simulink model "CDHRM_model_v1"  (R2019b)
settings: Solver=VariableStepAuto  StartTime=0.0  StopTime=10.0  RelTol=1e-3
InitFcn:
  | parameters.m
values from neighbouring files (symbols this model uses):
  a = 140/1000    (= 0.14)    [parameters.m]
  d = 23/2000    (= 0.0115)    [parameters.m]
  eta = 0.39    [parameters.m]
  g = 9.81    [parameters.m]
  J_L = 0.014 * 10e-7    (= 1.4e-08)    [parameters.m]
  J_R = 0.864 * 10e-7    (= 8.64e-07)    [parameters.m]
  k_m = 2560*100*pi/3    (= 268082.573106)    [parameters.m]
  k_trans = 0.36    [parameters.m]
  l_link = a-2*d    (= 0.117)    [parameters.m]
  m = 0.2    [parameters.m]
  mu_cable = 0.17    [parameters.m]
  n_0 = 9620*pi/30    (= 1007.40404425)    [parameters.m]
  p = 8/1000    (= 0.008)    [parameters.m]
  r = 20.5/1000    (= 0.0205)    [parameters.m]
  r_drum = 0.042    [parameters.m]
undefined symbols (not defined in the file or in its folder): d_drum
libraries: dspindex x18, dspinverses x1, simulink x1
(part 4 of 5)

== matlab function CDHRM_model_v1/Dynamic Model of the arm/M_inv(theta)/Newton-Euler Inverse Dynamics Block 11/Newton-Euler Recursive Inverse Dynamics Block ==
  data: theta input; u output; d_theta input; dd_theta input; m input; a input; d input; r input; g input; F_ec input; T_ec input
%% Neton-Euler Recursive Algorithm for Inverse Dynamics
function u  = fcn(theta, d_theta,dd_theta,m,a,d,r,g,F_ec,T_ec)
%% Parameters
N=9;
P_joint_to_joint=[a+2*d;0;0];
P_link_cm=[-(a/2+d);0;0];
z_0=[0;0;1];
x_0=[1;0;0];
% Create the D-H parameter table
DH_params=zeros(2*N,4);
for i=1:N
    if rem(i,2)==0
        DH_params(2*i-1:2*i,:)=[180+(theta(2*i-1)*180/pi) 90 0 0;...
                                180+(theta(2*i)*180/pi) 0 a 0];
    else
        DH_params(2*i-1:2*i,:)=[theta(2*i-1)*180/pi 90 0 0;...
                                theta(2*i)*180/pi 0 a 0];
    end
end
% Calculate transformation matrix n_A_n+1 (A_wrt_prev) and store in cell
% array
R = cell(2*N,1);
for n=1:2*N
    theta_i=DH_params(n,1);
    alpha_i=DH_params(n,2);
    R{n}=[cosd(theta_i) -sind(theta_i)*cosd(alpha_i) sind(theta_i)*sind(alpha_i);...
       sind(theta_i)  cosd(theta_i)*cosd(alpha_i) -cosd(theta_i)*sind(alpha_i);...
                  0              sind(alpha_i)   cosd(alpha_i) ];
end
% Calculate Inertia tensor
I = cell(N,1);
for i=1:N
    I{i}=[1/12*(m*(a)^2)+1/4*(m*r^2) 0 0;
                      0 1/12*(m*(a)^2)+1/4*(m*r^2) 0;
                      0 0 1/4*(m*r^2)];
end
%% Forward recursion
% Initialising the matrices
omega=zeros(3,N);
d_omega=zeros(3,N);
a_joint=zeros(3,N);
a_c=zeros(3,N);
% Initialising prev values
omega_prev=zeros(3,1);
d_omega_prev=zeros(3,1);
a_joint_prev=zeros(3,1);
for n=1:N
    omega(:,n)=(R{2*n-1}*R{2*n})'*(omega_prev + z_0*d_theta(2*n-1)) + ...
               (R{2*n})'*z_0*d_theta(2*n);
    d_omega(:,n)=(R{2*n-1}*R{2*n})'*(d_omega_prev + z_0*dd_theta(2*n-1)+...
                                     cross(omega(:,n),z_0*d_theta(2*n-1))) + ...
                 (R{2*n-1}*R{2*n})'*(cross((z_0*d_theta(2*n-1) + omega_prev),R{2*n-1}*z_0*d_theta(2*n))) + ...
                 (R{2*n})'*(z_0*dd_theta(2*n));
    if n==1
        a_joint(:,n)=[0;0;g];
    else
        a_joint(:,n)=(R{2*n-3}*R{2*n-2})'*a_joint_prev+ ...
                     cross(d_omega_prev,P_joint_to_joint)+...
                     cross(omega_prev,cross(omega_prev,P_joint_to_joint));
    end
    a_c(:,n)=(R{2*n-1}*R{2*n})'*a_joint(:,n)+...
             cross(d_omega(:,n),(P_joint_to_joint+P_link_cm))+...
             cross(omega(:,n),cross(omega(:,n),(P_joint_to_joint+P_link_cm)));
    % Update prev values for next iteration
    omega_prev=omega(:,n);
    d_omega_prev=d_omega(:,n);
    a_joint_prev=a_joint(:,n);
end

%% Backward recursion
% Initialising the matrices
F=zeros(3,N);
tau=zeros(3,N);
% Initialise next values
F_next=zeros(3,1);
tau_next=zeros(3,1);
for n=N:-1:1
   F(:,n) = F_next + m*a_c(:,n)-F_ec(:,n);
   tau(:,n) = tau_next - cross(F(:,n),(P_joint_to_joint+P_link_cm)) + ...
              cross(F_next,P_link_cm) + ...
              I{n}*d_omega(:,n)+ cross(omega(:,n),I{n}*omega(:,n))-T_ec(:,n);
   % Update next values for next iteration
   F_next=F(:,n);
   tau_next=tau(:,n);
end
%% Computing the output
u=vecnorm(tau)';

== matlab function CDHRM_model_v1/Dynamic Model of the arm/M_inv(theta)/Newton-Euler Inverse Dynamics Block 12/Cable Contact Forces ==
  data: tau_m input; theta input; a input; d input; r input; F_ec output; T_ec output; r_drum input; l_link input; eta input; mu input
function [F_ec,T_ec] = fcn(tau_m,theta,a,d,r,r_drum, l_link,eta,mu)
N=9;
F_ec=zeros(3,N);
T_ec=zeros(3,N);
F_cd=cell(N,3*N);
F_cp=cell(N,3*N);
for i=1:N
    for j=1:3*N
        F_cd{i,j}=[0;0;0];
        F_cp{i,j}=[0;0;0]; 
    end
end
r_d=cell(N,3*N);
r_p=cell(N,3*N);
T_p=cell(N,3*N);
T_d=cell(N,3*N);
P_link_cm=[-(a/2+d);0;0];
% Initialise prev values
Td_0=tau_m*r_drum/eta;
% Calculate the Transformation matrices
DH_params=zeros(2*N,4);
for i=1:N
    if rem(i,2)==0
        DH_params(2*i-1:2*i,:)=[180+(theta(2*i-1)*180/pi) 90 0 0; 180+(theta(2*i)*180/pi) 0 a 0];
    else
        DH_params(2*i-1:2*i,:)=[(theta(2*i-1)*180/pi) 90 0 0; (theta(2*i)*180/pi) 0 a 0];
    end
end

% Calculate transformation matrix n_A_n+1 (A_wrt_prev) and store in cell
% array
A = cell(2*N,1);
for n=1:2*N
    theta_i=DH_params(n,1);
    alpha_i=DH_params(n,2);
    r_i=DH_params(n,3);
    d_i=DH_params(n,4);
    A{n}=[cosd(theta_i) -sind(theta_i)*cosd(alpha_i) sind(theta_i)*sind(alpha_i) r_i*cosd(theta_i);...
       sind(theta_i)  cosd(theta_i)*cosd(alpha_i) -cosd(theta_i)*sind(alpha_i) r_i*sind(theta_i);...
                  0              sind(alpha_i)   cosd(alpha_i)              d_i;...
                  0              0              0                         1];
end

% Create a list of transformation matrices wrt base for all joints
A_wrt_base=cell(2*N,1);
A_wrt_base{1}=A{1};
for n=2:2*N
    A_wrt_base{n}=A_wrt_base{n-1}*A{n};
end

for i=1:N
    for j=1:3*N
        M=floor((j-1)/3)+1;
        if j==1
           Td_prev=Td_0(j);
        end
        % Calculate delta and r
        if rem(i,2)==0
            delta_p=((120/(N+1))*(M)+120*(j-1)+87);
            delta_d=((120/(N+1))*(M)+120*(j-1)-3);
            r_p_j=[d-l_link; r*cosd(delta_p);r*sind(delta_p); 1];
            r_d_j=[-d;r*cosd(delta_d);r*sind(delta_d); 1];
        else
            delta_p=((120/(N+1))*(M)+120*(j-1)-3);
            delta_d=((120/(N+1))*(M)+120*(j-1)+87);
            if i==1
                L_d_prev=[-d;r*cosd(delta_d);r*sind(delta_d); 1];
                e_d_prev=L_d_prev(1:3)/norm(L_d_prev(1:3));
                e_d_0=e_d_prev;
                r_d_prev=[-d;r*cosd(delta_d);r*sind(delta_d); 1];
            end
            r_p_j=[d-l_link; r*sind(delta_p);-r*cosd(delta_p); 1];
            r_d_j=[-d;r*sind(delta_d);-r*cosd(delta_d); 1];
        end
        r_p{i,j}=r_p_j(1:3);
        r_d{i,j}=r_d_j(1:3);
        % Calculate L
        if i==1
            L_p=(A{2*i}*r_p_j)-(r_d_prev);
        else
            L_p=(A{2*i}*r_p_j)-(A{2*i-2}*r_d_prev);
        end
        L_d=A{2*i}*(r_d_j-r_p_j);
        % Calculate e
        e_p=L_p(1:3)/norm(L_p(1:3));
        e_d=L_d(1:3)/norm(L_d(1:3));
        % Calculate phi
        phi_p=acos(dot(e_p,e_d));
        phi_d=acos(dot(e_d_prev,e_p));
        % Get Tp
        T_p_j=Td_prev/(exp(mu*phi_d));
        T_p{i,j}=T_p_j*e_p;
        % Get Td
        T_d_j=T_p_j/(exp(mu*phi_p));
        T_d{i,j}=T_d_j*e_d;
        % Update prev values
        e_d_prev=e_d;
        r_d_prev=r_d_j;
        Td_prev=T_d_j;
    end
end

% Calculate F_cp and F_cd
for n=1:N
    for k=1:3*N
        M=floor((k-1)/3)+1;
        if (3*n+1 <= k) && (k<=3*N) && n<=M
            F_cp{n,k}=T_d{n,k}-T_p{n,k};
            if n==1
                F_cd{n,k}=T_p{n,k}-((tau_m(k)*r_drum/eta)*e_d_0);
            else
                F_cd{n,k}=T_p{n,k}-T_d{n-1,k};
            end
        end
        if (3*n-2 <= k) && (k <=3*n) && n==M
            F_cp{n,k}=-T_p{n,k};
        end
    end
end

% Calculate F_ec
for n=1:N
    F_ec_n=[0;0;0];
    A_2n=inv(A{2*n});
    R_2n=A_2n(1:3,1:3);
    for k=3*n+1:3*N
        F_ec_n=F_ec_n+((R_2n)*F_cd{n,k});
    end
    for k=3*n-2:3*N
        F_ec_n=F_ec_n+((R_2n)*F_cp{n,k});
    end
    F_ec(:,n)=F_ec_n;
end

% Calculate T_ec
for n=1:N
    T_ec_n=[0;0;0];
    A_2n=inv(A{2*n});
    R_2n=A_2n(1:3,1:3);
    for k=3*n+1:3*N
        T_ec_n=T_ec_n+cross((r_d{n,k}-P_link_cm),((R_2n)*F_cd{n,k}));
    end
    for k=3*n-2:3*N
        T_ec_n=T_ec_n+cross((r_p{n,k}-P_link_cm),((R_2n)*F_cp{n,k}));
    end
    T_ec(:,n)=T_ec_n;
end

== matlab function CDHRM_model_v1/Dynamic Model of the arm/M_inv(theta)/Newton-Euler Inverse Dynamics Block 12/Newton-Euler Recursive Inverse Dynamics Block ==
  data: theta input; u output; d_theta input; dd_theta input; m input; a input; d input; r input; g input; F_ec input; T_ec input
%% Neton-Euler Recursive Algorithm for Inverse Dynamics
function u  = fcn(theta, d_theta,dd_theta,m,a,d,r,g,F_ec,T_ec)
%% Parameters
N=9;
P_joint_to_joint=[a+2*d;0;0];
P_link_cm=[-(a/2+d);0;0];
z_0=[0;0;1];
x_0=[1;0;0];
% Create the D-H parameter table
DH_params=zeros(2*N,4);
for i=1:N
    if rem(i,2)==0
        DH_params(2*i-1:2*i,:)=[180+(theta(2*i-1)*180/pi) 90 0 0;...
                                180+(theta(2*i)*180/pi) 0 a 0];
    else
        DH_params(2*i-1:2*i,:)=[theta(2*i-1)*180/pi 90 0 0;...
                                theta(2*i)*180/pi 0 a 0];
    end
end
% Calculate transformation matrix n_A_n+1 (A_wrt_prev) and store in cell
% array
R = cell(2*N,1);
for n=1:2*N
    theta_i=DH_params(n,1);
    alpha_i=DH_params(n,2);
    R{n}=[cosd(theta_i) -sind(theta_i)*cosd(alpha_i) sind(theta_i)*sind(alpha_i);...
       sind(theta_i)  cosd(theta_i)*cosd(alpha_i) -cosd(theta_i)*sind(alpha_i);...
                  0              sind(alpha_i)   cosd(alpha_i) ];
end
% Calculate Inertia tensor
I = cell(N,1);
for i=1:N
    I{i}=[1/12*(m*(a)^2)+1/4*(m*r^2) 0 0;
                      0 1/12*(m*(a)^2)+1/4*(m*r^2) 0;
                      0 0 1/4*(m*r^2)];
end
%% Forward recursion
% Initialising the matrices
omega=zeros(3,N);
d_omega=zeros(3,N);
a_joint=zeros(3,N);
a_c=zeros(3,N);
% Initialising prev values
omega_prev=zeros(3,1);
d_omega_prev=zeros(3,1);
a_joint_prev=zeros(3,1);
for n=1:N
    omega(:,n)=(R{2*n-1}*R{2*n})'*(omega_prev + z_0*d_theta(2*n-1)) + ...
               (R{2*n})'*z_0*d_theta(2*n);
    d_omega(:,n)=(R{2*n-1}*R{2*n})'*(d_omega_prev + z_0*dd_theta(2*n-1)+...
                                     cross(omega(:,n),z_0*d_theta(2*n-1))) + ...
                 (R{2*n-1}*R{2*n})'*(cross((z_0*d_theta(2*n-1) + omega_prev),R{2*n-1}*z_0*d_theta(2*n))) + ...
                 (R{2*n})'*(z_0*dd_theta(2*n));
    if n==1
        a_joint(:,n)=[0;0;g];
    else
        a_joint(:,n)=(R{2*n-3}*R{2*n-2})'*a_joint_prev+ ...
                     cross(d_omega_prev,P_joint_to_joint)+...
                     cross(omega_prev,cross(omega_prev,P_joint_to_joint));
    end
    a_c(:,n)=(R{2*n-1}*R{2*n})'*a_joint(:,n)+...
             cross(d_omega(:,n),(P_joint_to_joint+P_link_cm))+...
             cross(omega(:,n),cross(omega(:,n),(P_joint_to_joint+P_link_cm)));
    % Update prev values for next iteration
    omega_prev=omega(:,n);
    d_omega_prev=d_omega(:,n);
    a_joint_prev=a_joint(:,n);
end

%% Backward recursion
% Initialising the matrices
F=zeros(3,N);
tau=zeros(3,N);
% Initialise next values
F_next=zeros(3,1);
tau_next=zeros(3,1);
for n=N:-1:1
   F(:,n) = F_next + m*a_c(:,n)-F_ec(:,n);
   tau(:,n) = tau_next - cross(F(:,n),(P_joint_to_joint+P_link_cm)) + ...
              cross(F_next,P_link_cm) + ...
              I{n}*d_omega(:,n)+ cross(omega(:,n),I{n}*omega(:,n))-T_ec(:,n);
   % Update next values for next iteration
   F_next=F(:,n);
   tau_next=tau(:,n);
end
%% Computing the output
u=vecnorm(tau)';

== matlab function CDHRM_model_v1/Dynamic Model of the arm/M_inv(theta)/Newton-Euler Inverse Dynamics Block 13/Cable Contact Forces ==
  data: tau_m input; theta input; a input; d input; r input; F_ec output; T_ec output; r_drum input; l_link input; eta input; mu input
function [F_ec,T_ec] = fcn(tau_m,theta,a,d,r,r_drum, l_link,eta,mu)
N=9;
F_ec=zeros(3,N);
T_ec=zeros(3,N);
F_cd=cell(N,3*N);
F_cp=cell(N,3*N);
for i=1:N
    for j=1:3*N
        F_cd{i,j}=[0;0;0];
        F_cp{i,j}=[0;0;0]; 
    end
end
r_d=cell(N,3*N);
r_p=cell(N,3*N);
T_p=cell(N,3*N);
T_d=cell(N,3*N);
P_link_cm=[-(a/2+d);0;0];
% Initialise prev values
Td_0=tau_m*r_drum/eta;
% Calculate the Transformation matrices
DH_params=zeros(2*N,4);
for i=1:N
    if rem(i,2)==0
        DH_params(2*i-1:2*i,:)=[180+(theta(2*i-1)*180/pi) 90 0 0; 180+(theta(2*i)*180/pi) 0 a 0];
    else
        DH_params(2*i-1:2*i,:)=[(theta(2*i-1)*180/pi) 90 0 0; (theta(2*i)*180/pi) 0 a 0];
    end
end

% Calculate transformation matrix n_A_n+1 (A_wrt_prev) and store in cell
% array
A = cell(2*N,1);
for n=1:2*N
    theta_i=DH_params(n,1);
    alpha_i=DH_params(n,2);
    r_i=DH_params(n,3);
    d_i=DH_params(n,4);
    A{n}=[cosd(theta_i) -sind(theta_i)*cosd(alpha_i) sind(theta_i)*sind(alpha_i) r_i*cosd(theta_i);...
       sind(theta_i)  cosd(theta_i)*cosd(alpha_i) -cosd(theta_i)*sind(alpha_i) r_i*sind(theta_i);...
                  0              sind(alpha_i)   cosd(alpha_i)              d_i;...
                  0              0              0                         1];
end

% Create a list of transformation matrices wrt base for all joints
A_wrt_base=cell(2*N,1);
A_wrt_base{1}=A{1};
for n=2:2*N
    A_wrt_base{n}=A_wrt_base{n-1}*A{n};
end

for i=1:N
    for j=1:3*N
        M=floor((j-1)/3)+1;
        if j==1
           Td_prev=Td_0(j);
        end
        % Calculate delta and r
        if rem(i,2)==0
            delta_p=((120/(N+1))*(M)+120*(j-1)+87);
            delta_d=((120/(N+1))*(M)+120*(j-1)-3);
            r_p_j=[d-l_link; r*cosd(delta_p);r*sind(delta_p); 1];
            r_d_j=[-d;r*cosd(delta_d);r*sind(delta_d); 1];
        else
            delta_p=((120/(N+1))*(M)+120*(j-1)-3);
            delta_d=((120/(N+1))*(M)+120*(j-1)+87);
            if i==1
                L_d_prev=[-d;r*cosd(delta_d);r*sind(delta_d); 1];
                e_d_prev=L_d_prev(1:3)/norm(L_d_prev(1:3));
                e_d_0=e_d_prev;
                r_d_prev=[-d;r*cosd(delta_d);r*sind(delta_d); 1];
            end
            r_p_j=[d-l_link; r*sind(delta_p);-r*cosd(delta_p); 1];
            r_d_j=[-d;r*sind(delta_d);-r*cosd(delta_d); 1];
        end
        r_p{i,j}=r_p_j(1:3);
        r_d{i,j}=r_d_j(1:3);
        % Calculate L
        if i==1
            L_p=(A{2*i}*r_p_j)-(r_d_prev);
        else
            L_p=(A{2*i}*r_p_j)-(A{2*i-2}*r_d_prev);
        end
        L_d=A{2*i}*(r_d_j-r_p_j);
        % Calculate e
        e_p=L_p(1:3)/norm(L_p(1:3));
        e_d=L_d(1:3)/norm(L_d(1:3));
        % Calculate phi
        phi_p=acos(dot(e_p,e_d));
        phi_d=acos(dot(e_d_prev,e_p));
        % Get Tp
        T_p_j=Td_prev/(exp(mu*phi_d));
        T_p{i,j}=T_p_j*e_p;
        % Get Td
        T_d_j=T_p_j/(exp(mu*phi_p));
        T_d{i,j}=T_d_j*e_d;
        % Update prev values
        e_d_prev=e_d;
        r_d_prev=r_d_j;
        Td_prev=T_d_j;
    end
end

% Calculate F_cp and F_cd
for n=1:N
    for k=1:3*N
        M=floor((k-1)/3)+1;
        if (3*n+1 <= k) && (k<=3*N) && n<=M
            F_cp{n,k}=T_d{n,k}-T_p{n,k};
            if n==1
                F_cd{n,k}=T_p{n,k}-((tau_m(k)*r_drum/eta)*e_d_0);
            else
                F_cd{n,k}=T_p{n,k}-T_d{n-1,k};
            end
        end
        if (3*n-2 <= k) && (k <=3*n) && n==M
            F_cp{n,k}=-T_p{n,k};
        end
    end
end

% Calculate F_ec
for n=1:N
    F_ec_n=[0;0;0];
    A_2n=inv(A{2*n});
    R_2n=A_2n(1:3,1:3);
    for k=3*n+1:3*N
        F_ec_n=F_ec_n+((R_2n)*F_cd{n,k});
    end
    for k=3*n-2:3*N
        F_ec_n=F_ec_n+((R_2n)*F_cp{n,k});
    end
    F_ec(:,n)=F_ec_n;
end

% Calculate T_ec
for n=1:N
    T_ec_n=[0;0;0];
    A_2n=inv(A{2*n});
    R_2n=A_2n(1:3,1:3);
    for k=3*n+1:3*N
        T_ec_n=T_ec_n+cross((r_d{n,k}-P_link_cm),((R_2n)*F_cd{n,k}));
    end
    for k=3*n-2:3*N
        T_ec_n=T_ec_n+cross((r_p{n,k}-P_link_cm),((R_2n)*F_cp{n,k}));
    end
    T_ec(:,n)=T_ec_n;
end

== matlab function CDHRM_model_v1/Dynamic Model of the arm/M_inv(theta)/Newton-Euler Inverse Dynamics Block 13/Newton-Euler Recursive Inverse Dynamics Block ==
  data: theta input; u output; d_theta input; dd_theta input; m input; a input; d input; r input; g input; F_ec input; T_ec input
%% Neton-Euler Recursive Algorithm for Inverse Dynamics
function u  = fcn(theta, d_theta,dd_theta,m,a,d,r,g,F_ec,T_ec)
%% Parameters
N=9;
P_joint_to_joint=[a+2*d;0;0];
P_link_cm=[-(a/2+d);0;0];
z_0=[0;0;1];
x_0=[1;0;0];
% Create the D-H parameter table
DH_params=zeros(2*N,4);
for i=1:N
    if rem(i,2)==0
        DH_params(2*i-1:2*i,:)=[180+(theta(2*i-1)*180/pi) 90 0 0;...
                                180+(theta(2*i)*180/pi) 0 a 0];
    else
        DH_params(2*i-1:2*i,:)=[theta(2*i-1)*180/pi 90 0 0;...
                                theta(2*i)*180/pi 0 a 0];
    end
end
% Calculate transformation matrix n_A_n+1 (A_wrt_prev) and store in cell
% array
R = cell(2*N,1);
for n=1:2*N
    theta_i=DH_params(n,1);
    alpha_i=DH_params(n,2);
    R{n}=[cosd(theta_i) -sind(theta_i)*cosd(alpha_i) sind(theta_i)*sind(alpha_i);...
       sind(theta_i)  cosd(theta_i)*cosd(alpha_i) -cosd(theta_i)*sind(alpha_i);...
                  0              sind(alpha_i)   cosd(alpha_i) ];
end
% Calculate Inertia tensor
I = cell(N,1);
for i=1:N
    I{i}=[1/12*(m*(a)^2)+1/4*(m*r^2) 0 0;
                      0 1/12*(m*(a)^2)+1/4*(m*r^2) 0;
                      0 0 1/4*(m*r^2)];
end
%% Forward recursion
% Initialising the matrices
omega=zeros(3,N);
d_omega=zeros(3,N);
a_joint=zeros(3,N);
a_c=zeros(3,N);
% Initialising prev values
omega_prev=zeros(3,1);
d_omega_prev=zeros(3,1);
a_joint_prev=zeros(3,1);
for n=1:N
    omega(:,n)=(R{2*n-1}*R{2*n})'*(omega_prev + z_0*d_theta(2*n-1)) + ...
               (R{2*n})'*z_0*d_theta(2*n);
    d_omega(:,n)=(R{2*n-1}*R{2*n})'*(d_omega_prev + z_0*dd_theta(2*n-1)+...
                                     cross(omega(:,n),z_0*d_theta(2*n-1))) + ...
                 (R{2*n-1}*R{2*n})'*(cross((z_0*d_theta(2*n-1) + omega_prev),R{2*n-1}*z_0*d_theta(2*n))) + ...
                 (R{2*n})'*(z_0*dd_theta(2*n));
    if n==1
        a_joint(:,n)=[0;0;g];
    else
        a_joint(:,n)=(R{2*n-3}*R{2*n-2})'*a_joint_prev+ ...
                     cross(d_omega_prev,P_joint_to_joint)+...
                     cross(omega_prev,cross(omega_prev,P_joint_to_joint));
    end
    a_c(:,n)=(R{2*n-1}*R{2*n})'*a_joint(:,n)+...
             cross(d_omega(:,n),(P_joint_to_joint+P_link_cm))+...
             cross(omega(:,n),cross(omega(:,n),(P_joint_to_joint+P_link_cm)));
    % Update prev values for next iteration
    omega_prev=omega(:,n);
    d_omega_prev=d_omega(:,n);
    a_joint_prev=a_joint(:,n);
end

%% Backward recursion
% Initialising the matrices
F=zeros(3,N);
tau=zeros(3,N);
% Initialise next values
F_next=zeros(3,1);
tau_next=zeros(3,1);
for n=N:-1:1
   F(:,n) = F_next + m*a_c(:,n)-F_ec(:,n);
   tau(:,n) = tau_next - cross(F(:,n),(P_joint_to_joint+P_link_cm)) + ...
              cross(F_next,P_link_cm) + ...
              I{n}*d_omega(:,n)+ cross(omega(:,n),I{n}*omega(:,n))-T_ec(:,n);
   % Update next values for next iteration
   F_next=F(:,n);
   tau_next=tau(:,n);
end
%% Computing the output
u=vecnorm(tau)';

== matlab function CDHRM_model_v1/Dynamic Model of the arm/M_inv(theta)/Newton-Euler Inverse Dynamics Block 14/Cable Contact Forces ==
  data: tau_m input; theta input; a input; d input; r input; F_ec output; T_ec output; r_drum input; l_link input; eta input; mu input
function [F_ec,T_ec] = fcn(tau_m,theta,a,d,r,r_drum, l_link,eta,mu)
N=9;
F_ec=zeros(3,N);
T_ec=zeros(3,N);
F_cd=cell(N,3*N);
F_cp=cell(N,3*N);
for i=1:N
    for j=1:3*N
        F_cd{i,j}=[0;0;0];
        F_cp{i,j}=[0;0;0]; 
    end
end
r_d=cell(N,3*N);
r_p=cell(N,3*N);
T_p=cell(N,3*N);
T_d=cell(N,3*N);
P_link_cm=[-(a/2+d);0;0];
% Initialise prev values
Td_0=tau_m*r_drum/eta;
% Calculate the Transformation matrices
DH_params=zeros(2*N,4);
for i=1:N
    if rem(i,2)==0
        DH_params(2*i-1:2*i,:)=[180+(theta(2*i-1)*180/pi) 90 0 0; 180+(theta(2*i)*180/pi) 0 a 0];
    else
        DH_params(2*i-1:2*i,:)=[(theta(2*i-1)*180/pi) 90 0 0; (theta(2*i)*180/pi) 0 a 0];
    end
end

% Calculate transformation matrix n_A_n+1 (A_wrt_prev) and store in cell
% array
A = cell(2*N,1);
for n=1:2*N
    theta_i=DH_params(n,1);
    alpha_i=DH_params(n,2);
    r_i=DH_params(n,3);
    d_i=DH_params(n,4);
    A{n}=[cosd(theta_i) -sind(theta_i)*cosd(alpha_i) sind(theta_i)*sind(alpha_i) r_i*cosd(theta_i);...
       sind(theta_i)  cosd(theta_i)*cosd(alpha_i) -cosd(theta_i)*sind(alpha_i) r_i*sind(theta_i);...
                  0              sind(alpha_i)   cosd(alpha_i)              d_i;...
                  0              0              0                         1];
end

% Create a list of transformation matrices wrt base for all joints
A_wrt_base=cell(2*N,1);
A_wrt_base{1}=A{1};
for n=2:2*N
    A_wrt_base{n}=A_wrt_base{n-1}*A{n};
end

for i=1:N
    for j=1:3*N
        M=floor((j-1)/3)+1;
        if j==1
           Td_prev=Td_0(j);
        end
        % Calculate delta and r
        if rem(i,2)==0
            delta_p=((120/(N+1))*(M)+120*(j-1)+87);
            delta_d=((120/(N+1))*(M)+120*(j-1)-3);
            r_p_j=[d-l_link; r*cosd(delta_p);r*sind(delta_p); 1];
            r_d_j=[-d;r*cosd(delta_d);r*sind(delta_d); 1];
        else
            delta_p=((120/(N+1))*(M)+120*(j-1)-3);
            delta_d=((120/(N+1))*(M)+120*(j-1)+87);
            if i==1
                L_d_prev=[-d;r*cosd(delta_d);r*sind(delta_d); 1];
                e_d_prev=L_d_prev(1:3)/norm(L_d_prev(1:3));
                e_d_0=e_d_prev;
                r_d_prev=[-d;r*cosd(delta_d);r*sind(delta_d); 1];
            end
            r_p_j=[d-l_link; r*sind(delta_p);-r*cosd(delta_p); 1];
            r_d_j=[-d;r*sind(delta_d);-r*cosd(delta_d); 1];
        end
        r_p{i,j}=r_p_j(1:3);
        r_d{i,j}=r_d_j(1:3);
        % Calculate L
        if i==1
            L_p=(A{2*i}*r_p_j)-(r_d_prev);
        else
            L_p=(A{2*i}*r_p_j)-(A{2*i-2}*r_d_prev);
        end
        L_d=A{2*i}*(r_d_j-r_p_j);
        % Calculate e
        e_p=L_p(1:3)/norm(L_p(1:3));
        e_d=L_d(1:3)/norm(L_d(1:3));
        % Calculate phi
        phi_p=acos(dot(e_p,e_d));
        phi_d=acos(dot(e_d_prev,e_p));
        % Get Tp
        T_p_j=Td_prev/(exp(mu*phi_d));
        T_p{i,j}=T_p_j*e_p;
        % Get Td
        T_d_j=T_p_j/(exp(mu*phi_p));
        T_d{i,j}=T_d_j*e_d;
        % Update prev values
        e_d_prev=e_d;
        r_d_prev=r_d_j;
        Td_prev=T_d_j;
    end
end

% Calculate F_cp and F_cd
for n=1:N
    for k=1:3*N
        M=floor((k-1)/3)+1;
        if (3*n+1 <= k) && (k<=3*N) && n<=M
            F_cp{n,k}=T_d{n,k}-T_p{n,k};
            if n==1
                F_cd{n,k}=T_p{n,k}-((tau_m(k)*r_drum/eta)*e_d_0);
            else
                F_cd{n,k}=T_p{n,k}-T_d{n-1,k};
            end
        end
        if (3*n-2 <= k) && (k <=3*n) && n==M
            F_cp{n,k}=-T_p{n,k};
        end
    end
end

% Calculate F_ec
for n=1:N
    F_ec_n=[0;0;0];
    A_2n=inv(A{2*n});
    R_2n=A_2n(1:3,1:3);
    for k=3*n+1:3*N
        F_ec_n=F_ec_n+((R_2n)*F_cd{n,k});
    end
    for k=3*n-2:3*N
        F_ec_n=F_ec_n+((R_2n)*F_cp{n,k});
    end
    F_ec(:,n)=F_ec_n;
end

% Calculate T_ec
for n=1:N
    T_ec_n=[0;0;0];
    A_2n=inv(A{2*n});
    R_2n=A_2n(1:3,1:3);
    for k=3*n+1:3*N
        T_ec_n=T_ec_n+cross((r_d{n,k}-P_link_cm),((R_2n)*F_cd{n,k}));
    end
    for k=3*n-2:3*N
        T_ec_n=T_ec_n+cross((r_p{n,k}-P_link_cm),((R_2n)*F_cp{n,k}));
    end
    T_ec(:,n)=T_ec_n;
end

== matlab function CDHRM_model_v1/Dynamic Model of the arm/M_inv(theta)/Newton-Euler Inverse Dynamics Block 14/Newton-Euler Recursive Inverse Dynamics Block ==
  data: theta input; u output; d_theta input; dd_theta input; m input; a input; d input; r input; g input; F_ec input; T_ec input
%% Neton-Euler Recursive Algorithm for Inverse Dynamics
function u  = fcn(theta, d_theta,dd_theta,m,a,d,r,g,F_ec,T_ec)
%% Parameters
N=9;
P_joint_to_joint=[a+2*d;0;0];
P_link_cm=[-(a/2+d);0;0];
z_0=[0;0;1];
x_0=[1;0;0];
% Create the D-H parameter table
DH_params=zeros(2*N,4);
for i=1:N
    if rem(i,2)==0
        DH_params(2*i-1:2*i,:)=[180+(theta(2*i-1)*180/pi) 90 0 0;...
                                180+(theta(2*i)*180/pi) 0 a 0];
    else
        DH_params(2*i-1:2*i,:)=[theta(2*i-1)*180/pi 90 0 0;...
                                theta(2*i)*180/pi 0 a 0];
    end
end
% Calculate transformation matrix n_A_n+1 (A_wrt_prev) and store in cell
% array
R = cell(2*N,1);
for n=1:2*N
    theta_i=DH_params(n,1);
    alpha_i=DH_params(n,2);
    R{n}=[cosd(theta_i) -sind(theta_i)*cosd(alpha_i) sind(theta_i)*sind(alpha_i);...
       sind(theta_i)  cosd(theta_i)*cosd(alpha_i) -cosd(theta_i)*sind(alpha_i);...
                  0              sind(alpha_i)   cosd(alpha_i) ];
end
% Calculate Inertia tensor
I = cell(N,1);
for i=1:N
    I{i}=[1/12*(m*(a)^2)+1/4*(m*r^2) 0 0;
                      0 1/12*(m*(a)^2)+1/4*(m*r^2) 0;
                      0 0 1/4*(m*r^2)];
end
%% Forward recursion
% Initialising the matrices
omega=zeros(3,N);
d_omega=zeros(3,N);
a_joint=zeros(3,N);
a_c=zeros(3,N);
% Initialising prev values
omega_prev=zeros(3,1);
d_omega_prev=zeros(3,1);
a_joint_prev=zeros(3,1);
for n=1:N
    omega(:,n)=(R{2*n-1}*R{2*n})'*(omega_prev + z_0*d_theta(2*n-1)) + ...
               (R{2*n})'*z_0*d_theta(2*n);
    d_omega(:,n)=(R{2*n-1}*R{2*n})'*(d_omega_prev + z_0*dd_theta(2*n-1)+...
                                     cross(omega(:,n),z_0*d_theta(2*n-1))) + ...
                 (R{2*n-1}*R{2*n})'*(cross((z_0*d_theta(2*n-1) + omega_prev),R{2*n-1}*z_0*d_theta(2*n))) + ...
                 (R{2*n})'*(z_0*dd_theta(2*n));
    if n==1
        a_joint(:,n)=[0;0;g];
    else
        a_joint(:,n)=(R{2*n-3}*R{2*n-2})'*a_joint_prev+ ...
                     cross(d_omega_prev,P_joint_to_joint)+...
                     cross(omega_prev,cross(omega_prev,P_joint_to_joint));
    end
    a_c(:,n)=(R{2*n-1}*R{2*n})'*a_joint(:,n)+...
             cross(d_omega(:,n),(P_joint_to_joint+P_link_cm))+...
             cross(omega(:,n),cross(omega(:,n),(P_joint_to_joint+P_link_cm)));
    % Update prev values for next iteration
    omega_prev=omega(:,n);
    d_omega_prev=d_omega(:,n);
    a_joint_prev=a_joint(:,n);
end

%% Backward recursion
% Initialising the matrices
F=zeros(3,N);
tau=zeros(3,N);
% Initialise next values
F_next=zeros(3,1);
tau_next=zeros(3,1);
for n=N:-1:1
   F(:,n) = F_next + m*a_c(:,n)-F_ec(:,n);
   tau(:,n) = tau_next - cross(F(:,n),(P_joint_to_joint+P_link_cm)) + ...
              cross(F_next,P_link_cm) + ...
              I{n}*d_omega(:,n)+ cross(omega(:,n),I{n}*omega(:,n))-T_ec(:,n);
   % Update next values for next iteration
   F_next=F(:,n);
   tau_next=tau(:,n);
end
%% Computing the output
u=vecnorm(tau)';

== matlab function CDHRM_model_v1/Dynamic Model of the arm/M_inv(theta)/Newton-Euler Inverse Dynamics Block 15/Cable Contact Forces ==
  data: tau_m input; theta input; a input; d input; r input; F_ec output; T_ec output; r_drum input; l_link input; eta input; mu input
function [F_ec,T_ec] = fcn(tau_m,theta,a,d,r,r_drum, l_link,eta,mu)
N=9;
F_ec=zeros(3,N);
T_ec=zeros(3,N);
F_cd=cell(N,3*N);
F_cp=cell(N,3*N);
for i=1:N
    for j=1:3*N
        F_cd{i,j}=[0;0;0];
        F_cp{i,j}=[0;0;0]; 
    end
end
r_d=cell(N,3*N);
r_p=cell(N,3*N);
T_p=cell(N,3*N);
T_d=cell(N,3*N);
P_link_cm=[-(a/2+d);0;0];
% Initialise prev values
Td_0=tau_m*r_drum/eta;
% Calculate the Transformation matrices
DH_params=zeros(2*N,4);
for i=1:N
    if rem(i,2)==0
        DH_params(2*i-1:2*i,:)=[180+(theta(2*i-1)*180/pi) 90 0 0; 180+(theta(2*i)*180/pi) 0 a 0];
    else
        DH_params(2*i-1:2*i,:)=[(theta(2*i-1)*180/pi) 90 0 0; (theta(2*i)*180/pi) 0 a 0];
    end
end

% Calculate transformation matrix n_A_n+1 (A_wrt_prev) and store in cell
% array
A = cell(2*N,1);
for n=1:2*N
    theta_i=DH_params(n,1);
    alpha_i=DH_params(n,2);
    r_i=DH_params(n,3);
    d_i=DH_params(n,4);
    A{n}=[cosd(theta_i) -sind(theta_i)*cosd(alpha_i) sind(theta_i)*sind(alpha_i) r_i*cosd(theta_i);...
       sind(theta_i)  cosd(theta_i)*cosd(alpha_i) -cosd(theta_i)*sind(alpha_i) r_i*sind(theta_i);...
                  0              sind(alpha_i)   cosd(alpha_i)              d_i;...
                  0              0              0                         1];
end

% Create a list of transformation matrices wrt base for all joints
A_wrt_base=cell(2*N,1);
A_wrt_base{1}=A{1};
for n=2:2*N
    A_wrt_base{n}=A_wrt_base{n-1}*A{n};
end

for i=1:N
    for j=1:3*N
        M=floor((j-1)/3)+1;
        if j==1
           Td_prev=Td_0(j);
        end
        % Calculate delta and r
        if rem(i,2)==0
            delta_p=((120/(N+1))*(M)+120*(j-1)+87);
            delta_d=((120/(N+1))*(M)+120*(j-1)-3);
            r_p_j=[d-l_link; r*cosd(delta_p);r*sind(delta_p); 1];
            r_d_j=[-d;r*cosd(delta_d);r*sind(delta_d); 1];
        else
            delta_p=((120/(N+1))*(M)+120*(j-1)-3);
            delta_d=((120/(N+1))*(M)+120*(j-1)+87);
            if i==1
                L_d_prev=[-d;r*cosd(delta_d);r*sind(delta_d); 1];
                e_d_prev=L_d_prev(1:3)/norm(L_d_prev(1:3));
                e_d_0=e_d_prev;
                r_d_prev=[-d;r*cosd(delta_d);r*sind(delta_d); 1];
            end
            r_p_j=[d-l_link; r*sind(delta_p);-r*cosd(delta_p); 1];
            r_d_j=[-d;r*sind(delta_d);-r*cosd(delta_d); 1];
        end
        r_p{i,j}=r_p_j(1:3);
        r_d{i,j}=r_d_j(1:3);
        % Calculate L
        if i==1
            L_p=(A{2*i}*r_p_j)-(r_d_prev);
        else
            L_p=(A{2*i}*r_p_j)-(A{2*i-2}*r_d_prev);
        end
        L_d=A{2*i}*(r_d_j-r_p_j);
        % Calculate e
        e_p=L_p(1:3)/norm(L_p(1:3));
        e_d=L_d(1:3)/norm(L_d(1:3));
        % Calculate phi
        phi_p=acos(dot(e_p,e_d));
        phi_d=acos(dot(e_d_prev,e_p));
        % Get Tp
        T_p_j=Td_prev/(exp(mu*phi_d));
        T_p{i,j}=T_p_j*e_p;
        % Get Td
        T_d_j=T_p_j/(exp(mu*phi_p));
        T_d{i,j}=T_d_j*e_d;
        % Update prev values
        e_d_prev=e_d;
        r_d_prev=r_d_j;
        Td_prev=T_d_j;
    end
end

% Calculate F_cp and F_cd
for n=1:N
    for k=1:3*N
        M=floor((k-1)/3)+1;
        if (3*n+1 <= k) && (k<=3*N) && n<=M
            F_cp{n,k}=T_d{n,k}-T_p{n,k};
            if n==1
                F_cd{n,k}=T_p{n,k}-((tau_m(k)*r_drum/eta)*e_d_0);
            else
                F_cd{n,k}=T_p{n,k}-T_d{n-1,k};
            end
        end
        if (3*n-2 <= k) && (k <=3*n) && n==M
            F_cp{n,k}=-T_p{n,k};
        end
    end
end

% Calculate F_ec
for n=1:N
    F_ec_n=[0;0;0];
    A_2n=inv(A{2*n});
    R_2n=A_2n(1:3,1:3);
    for k=3*n+1:3*N
        F_ec_n=F_ec_n+((R_2n)*F_cd{n,k});
    end
    for k=3*n-2:3*N
        F_ec_n=F_ec_n+((R_2n)*F_cp{n,k});
    end
    F_ec(:,n)=F_ec_n;
end

% Calculate T_ec
for n=1:N
    T_ec_n=[0;0;0];
    A_2n=inv(A{2*n});
    R_2n=A_2n(1:3,1:3);
    for k=3*n+1:3*N
        T_ec_n=T_ec_n+cross((r_d{n,k}-P_link_cm),((R_2n)*F_cd{n,k}));
    end
    for k=3*n-2:3*N
        T_ec_n=T_ec_n+cross((r_p{n,k}-P_link_cm),((R_2n)*F_cp{n,k}));
    end
    T_ec(:,n)=T_ec_n;
end

== matlab function CDHRM_model_v1/Dynamic Model of the arm/M_inv(theta)/Newton-Euler Inverse Dynamics Block 15/Newton-Euler Recursive Inverse Dynamics Block ==
  data: theta input; u output; d_theta input; dd_theta input; m input; a input; d input; r input; g input; F_ec input; T_ec input
%% Neton-Euler Recursive Algorithm for Inverse Dynamics
function u  = fcn(theta, d_theta,dd_theta,m,a,d,r,g,F_ec,T_ec)
%% Parameters
N=9;
P_joint_to_joint=[a+2*d;0;0];
P_link_cm=[-(a/2+d);0;0];
z_0=[0;0;1];
x_0=[1;0;0];
% Create the D-H parameter table
DH_params=zeros(2*N,4);
for i=1:N
    if rem(i,2)==0
        DH_params(2*i-1:2*i,:)=[180+(theta(2*i-1)*180/pi) 90 0 0;...
                                180+(theta(2*i)*180/pi) 0 a 0];
    else
        DH_params(2*i-1:2*i,:)=[theta(2*i-1)*180/pi 90 0 0;...
                                theta(2*i)*180/pi 0 a 0];
    end
end
% Calculate transformation matrix n_A_n+1 (A_wrt_prev) and store in cell
% array
R = cell(2*N,1);
for n=1:2*N
    theta_i=DH_params(n,1);
    alpha_i=DH_params(n,2);
    R{n}=[cosd(theta_i) -sind(theta_i)*cosd(alpha_i) sind(theta_i)*sind(alpha_i);...
       sind(theta_i)  cosd(theta_i)*cosd(alpha_i) -cosd(theta_i)*sind(alpha_i);...
                  0              sind(alpha_i)   cosd(alpha_i) ];
end
% Calculate Inertia tensor
I = cell(N,1);
for i=1:N
    I{i}=[1/12*(m*(a)^2)+1/4*(m*r^2) 0 0;
                      0 1/12*(m*(a)^2)+1/4*(m*r^2) 0;
                      0 0 1/4*(m*r^2)];
end
%% Forward recursion
% Initialising the matrices
omega=zeros(3,N);
d_omega=zeros(3,N);
a_joint=zeros(3,N);
a_c=zeros(3,N);
% Initialising prev values
omega_prev=zeros(3,1);
d_omega_prev=zeros(3,1);
a_joint_prev=zeros(3,1);
for n=1:N
    omega(:,n)=(R{2*n-1}*R{2*n})'*(omega_prev + z_0*d_theta(2*n-1)) + ...
               (R{2*n})'*z_0*d_theta(2*n);
    d_omega(:,n)=(R{2*n-1}*R{2*n})'*(d_omega_prev + z_0*dd_theta(2*n-1)+...
                                     cross(omega(:,n),z_0*d_theta(2*n-1))) + ...
                 (R{2*n-1}*R{2*n})'*(cross((z_0*d_theta(2*n-1) + omega_prev),R{2*n-1}*z_0*d_theta(2*n))) + ...
                 (R{2*n})'*(z_0*dd_theta(2*n));
    if n==1
        a_joint(:,n)=[0;0;g];
    else
        a_joint(:,n)=(R{2*n-3}*R{2*n-2})'*a_joint_prev+ ...
                     cross(d_omega_prev,P_joint_to_joint)+...
                     cross(omega_prev,cross(omega_prev,P_joint_to_joint));
    end
    a_c(:,n)=(R{2*n-1}*R{2*n})'*a_joint(:,n)+...
             cross(d_omega(:,n),(P_joint_to_joint+P_link_cm))+...
             cross(omega(:,n),cross(omega(:,n),(P_joint_to_joint+P_link_cm)));
    % Update prev values for next iteration
    omega_prev=omega(:,n);
    d_omega_prev=d_omega(:,n);
    a_joint_prev=a_joint(:,n);
end

%% Backward recursion
% Initialising the matrices
F=zeros(3,N);
tau=zeros(3,N);
% Initialise next values
F_next=zeros(3,1);
tau_next=zeros(3,1);
for n=N:-1:1
   F(:,n) = F_next + m*a_c(:,n)-F_ec(:,n);
   tau(:,n) = tau_next - cross(F(:,n),(P_joint_to_joint+P_link_cm)) + ...
              cross(F_next,P_link_cm) + ...
              I{n}*d_omega(:,n)+ cross(omega(:,n),I{n}*omega(:,n))-T_ec(:,n);
   % Update next values for next iteration
   F_next=F(:,n);
   tau_next=tau(:,n);
end
%% Computing the output
u=vecnorm(tau)';

== matlab function CDHRM_model_v1/Dynamic Model of the arm/M_inv(theta)/Newton-Euler Inverse Dynamics Block 16/Cable Contact Forces ==
  data: tau_m input; theta input; a input; d input; r input; F_ec output; T_ec output; r_drum input; l_link input; eta input; mu input
function [F_ec,T_ec] = fcn(tau_m,theta,a,d,r,r_drum, l_link,eta,mu)
N=9;
F_ec=zeros(3,N);
T_ec=zeros(3,N);
F_cd=cell(N,3*N);
F_cp=cell(N,3*N);
for i=1:N
    for j=1:3*N
        F_cd{i,j}=[0;0;0];
        F_cp{i,j}=[0;0;0]; 
    end
end
r_d=cell(N,3*N);
r_p=cell(N,3*N);
T_p=cell(N,3*N);
T_d=cell(N,3*N);
P_link_cm=[-(a/2+d);0;0];
% Initialise prev values
Td_0=tau_m*r_drum/eta;
% Calculate the Transformation matrices
DH_params=zeros(2*N,4);
for i=1:N
    if rem(i,2)==0
        DH_params(2*i-1:2*i,:)=[180+(theta(2*i-1)*180/pi) 90 0 0; 180+(theta(2*i)*180/pi) 0 a 0];
    else
        DH_params(2*i-1:2*i,:)=[(theta(2*i-1)*180/pi) 90 0 0; (theta(2*i)*180/pi) 0 a 0];
    end
end

% Calculate transformation matrix n_A_n+1 (A_wrt_prev) and store in cell
% array
A = cell(2*N,1);
for n=1:2*N
    theta_i=DH_params(n,1);
    alpha_i=DH_params(n,2);
    r_i=DH_params(n,3);
    d_i=DH_params(n,4);
    A{n}=[cosd(theta_i) -sind(theta_i)*cosd(alpha_i) sind(theta_i)*sind(alpha_i) r_i*cosd(theta_i);...
       sind(theta_i)  cosd(theta_i)*cosd(alpha_i) -cosd(theta_i)*sind(alpha_i) r_i*sind(theta_i);...
                  0              sind(alpha_i)   cosd(alpha_i)              d_i;...
                  0              0              0                         1];
end

% Create a list of transformation matrices wrt base for all joints
A_wrt_base=cell(2*N,1);
A_wrt_base{1}=A{1};
for n=2:2*N
    A_wrt_base{n}=A_wrt_base{n-1}*A{n};
end

for i=1:N
    for j=1:3*N
        M=floor((j-1)/3)+1;
        if j==1
           Td_prev=Td_0(j);
        end
        % Calculate delta and r
        if rem(i,2)==0
            delta_p=((120/(N+1))*(M)+120*(j-1)+87);
            delta_d=((120/(N+1))*(M)+120*(j-1)-3);
            r_p_j=[d-l_link; r*cosd(delta_p);r*sind(delta_p); 1];
            r_d_j=[-d;r*cosd(delta_d);r*sind(delta_d); 1];
        else
            delta_p=((120/(N+1))*(M)+120*(j-1)-3);
            delta_d=((120/(N+1))*(M)+120*(j-1)+87);
            if i==1
                L_d_prev=[-d;r*cosd(delta_d);r*sind(delta_d); 1];
                e_d_prev=L_d_prev(1:3)/norm(L_d_prev(1:3));
                e_d_0=e_d_prev;
                r_d_prev=[-d;r*cosd(delta_d);r*sind(delta_d); 1];
            end
            r_p_j=[d-l_link; r*sind(delta_p);-r*cosd(delta_p); 1];
            r_d_j=[-d;r*sind(delta_d);-r*cosd(delta_d); 1];
        end
        r_p{i,j}=r_p_j(1:3);
        r_d{i,j}=r_d_j(1:3);
        % Calculate L
        if i==1
            L_p=(A{2*i}*r_p_j)-(r_d_prev);
        else
            L_p=(A{2*i}*r_p_j)-(A{2*i-2}*r_d_prev);
        end
        L_d=A{2*i}*(r_d_j-r_p_j);
        % Calculate e
        e_p=L_p(1:3)/norm(L_p(1:3));
        e_d=L_d(1:3)/norm(L_d(1:3));
        % Calculate phi
        phi_p=acos(dot(e_p,e_d));
        phi_d=acos(dot(e_d_prev,e_p));
        % Get Tp
        T_p_j=Td_prev/(exp(mu*phi_d));
        T_p{i,j}=T_p_j*e_p;
        % Get Td
        T_d_j=T_p_j/(exp(mu*phi_p));
        T_d{i,j}=T_d_j*e_d;
        % Update prev values
        e_d_prev=e_d;
        r_d_prev=r_d_j;
        Td_prev=T_d_j;
    end
end

% Calculate F_cp and F_cd
for n=1:N
    for k=1:3*N
        M=floor((k-1)/3)+1;
        if (3*n+1 <= k) && (k<=3*N) && n<=M
            F_cp{n,k}=T_d{n,k}-T_p{n,k};
            if n==1
                F_cd{n,k}=T_p{n,k}-((tau_m(k)*r_drum/eta)*e_d_0);
            else
                F_cd{n,k}=T_p{n,k}-T_d{n-1,k};
            end
        end
        if (3*n-2 <= k) && (k <=3*n) && n==M
            F_cp{n,k}=-T_p{n,k};
        end
    end
end

% Calculate F_ec
for n=1:N
    F_ec_n=[0;0;0];
    A_2n=inv(A{2*n});
    R_2n=A_2n(1:3,1:3);
    for k=3*n+1:3*N
        F_ec_n=F_ec_n+((R_2n)*F_cd{n,k});
    end
    for k=3*n-2:3*N
        F_ec_n=F_ec_n+((R_2n)*F_cp{n,k});
    end
    F_ec(:,n)=F_ec_n;
end

% Calculate T_ec
for n=1:N
    T_ec_n=[0;0;0];
    A_2n=inv(A{2*n});
    R_2n=A_2n(1:3,1:3);
    for k=3*n+1:3*N
        T_ec_n=T_ec_n+cross((r_d{n,k}-P_link_cm),((R_2n)*F_cd{n,k}));
    end
    for k=3*n-2:3*N
        T_ec_n=T_ec_n+cross((r_p{n,k}-P_link_cm),((R_2n)*F_cp{n,k}));
    end
    T_ec(:,n)=T_ec_n;
end

== matlab function CDHRM_model_v1/Dynamic Model of the arm/M_inv(theta)/Newton-Euler Inverse Dynamics Block 16/Newton-Euler Recursive Inverse Dynamics Block ==
  data: theta input; u output; d_theta input; dd_theta input; m input; a input; d input; r input; g input; F_ec input; T_ec input
%% Neton-Euler Recursive Algorithm for Inverse Dynamics
function u  = fcn(theta, d_theta,dd_theta,m,a,d,r,g,F_ec,T_ec)
%% Parameters
N=9;
P_joint_to_joint=[a+2*d;0;0];
P_link_cm=[-(a/2+d);0;0];
z_0=[0;0;1];
x_0=[1;0;0];
% Create the D-H parameter table
DH_params=zeros(2*N,4);
for i=1:N
    if rem(i,2)==0
        DH_params(2*i-1:2*i,:)=[180+(theta(2*i-1)*180/pi) 90 0 0;...
                                180+(theta(2*i)*180/pi) 0 a 0];
    else
        DH_params(2*i-1:2*i,:)=[theta(2*i-1)*180/pi 90 0 0;...
                                theta(2*i)*180/pi 0 a 0];
    end
end
% Calculate transformation matrix n_A_n+1 (A_wrt_prev) and store in cell
% array
R = cell(2*N,1);
for n=1:2*N
    theta_i=DH_params(n,1);
    alpha_i=DH_params(n,2);
    R{n}=[cosd(theta_i) -sind(theta_i)*cosd(alpha_i) sind(theta_i)*sind(alpha_i);...
       sind(theta_i)  cosd(theta_i)*cosd(alpha_i) -cosd(theta_i)*sind(alpha_i);...
                  0              sind(alpha_i)   cosd(alpha_i) ];
end
% Calculate Inertia tensor
I = cell(N,1);
for i=1:N
    I{i}=[1/12*(m*(a)^2)+1/4*(m*r^2) 0 0;
                      0 1/12*(m*(a)^2)+1/4*(m*r^2) 0;
                      0 0 1/4*(m*r^2)];
end
%% Forward recursion
% Initialising the matrices
omega=zeros(3,N);
d_omega=zeros(3,N);
a_joint=zeros(3,N);
a_c=zeros(3,N);
% Initialising prev values
omega_prev=zeros(3,1);
d_omega_prev=zeros(3,1);
a_joint_prev=zeros(3,1);
for n=1:N
    omega(:,n)=(R{2*n-1}*R{2*n})'*(omega_prev + z_0*d_theta(2*n-1)) + ...
               (R{2*n})'*z_0*d_theta(2*n);
    d_omega(:,n)=(R{2*n-1}*R{2*n})'*(d_omega_prev + z_0*dd_theta(2*n-1)+...
                                     cross(omega(:,n),z_0*d_theta(2*n-1))) + ...
                 (R{2*n-1}*R{2*n})'*(cross((z_0*d_theta(2*n-1) + omega_prev),R{2*n-1}*z_0*d_theta(2*n))) + ...
                 (R{2*n})'*(z_0*dd_theta(2*n));
    if n==1
        a_joint(:,n)=[0;0;g];
    else
        a_joint(:,n)=(R{2*n-3}*R{2*n-2})'*a_joint_prev+ ...
                     cross(d_omega_prev,P_joint_to_joint)+...
                     cross(omega_prev,cross(omega_prev,P_joint_to_joint));
    end
    a_c(:,n)=(R{2*n-1}*R{2*n})'*a_joint(:,n)+...
             cross(d_omega(:,n),(P_joint_to_joint+P_link_cm))+...
             cross(omega(:,n),cross(omega(:,n),(P_joint_to_joint+P_link_cm)));
    % Update prev values for next iteration
    omega_prev=omega(:,n);
    d_omega_prev=d_omega(:,n);
    a_joint_prev=a_joint(:,n);
end

%% Backward recursion
% Initialising the matrices
F=zeros(3,N);
tau=zeros(3,N);
% Initialise next values
F_next=zeros(3,1);
tau_next=zeros(3,1);
for n=N:-1:1
   F(:,n) = F_next + m*a_c(:,n)-F_ec(:,n);
   tau(:,n) = tau_next - cross(F(:,n),(P_joint_to_joint+P_link_cm)) + ...
              cross(F_next,P_link_cm) + ...
              I{n}*d_omega(:,n)+ cross(omega(:,n),I{n}*omega(:,n))-T_ec(:,n);
   % Update next values for next iteration
   F_next=F(:,n);
   tau_next=tau(:,n);
end
%% Computing the output
u=vecnorm(tau)';

== matlab function CDHRM_model_v1/Dynamic Model of the arm/M_inv(theta)/Newton-Euler Inverse Dynamics Block 17/Cable Contact Forces ==
  data: tau_m input; theta input; a input; d input; r input; F_ec output; T_ec output; r_drum input; l_link input; eta input; mu input
function [F_ec,T_ec] = fcn(tau_m,theta,a,d,r,r_drum, l_link,eta,mu)
N=9;
F_ec=zeros(3,N);
T_ec=zeros(3,N);
F_cd=cell(N,3*N);
F_cp=cell(N,3*N);
for i=1:N
    for j=1:3*N
        F_cd{i,j}=[0;0;0];
        F_cp{i,j}=[0;0;0]; 
    end
end
r_d=cell(N,3*N);
r_p=cell(N,3*N);
T_p=cell(N,3*N);
T_d=cell(N,3*N);
P_link_cm=[-(a/2+d);0;0];
% Initialise prev values
Td_0=tau_m*r_drum/eta;
% Calculate the Transformation matrices
DH_params=zeros(2*N,4);
for i=1:N
    if rem(i,2)==0
        DH_params(2*i-1:2*i,:)=[180+(theta(2*i-1)*180/pi) 90 0 0; 180+(theta(2*i)*180/pi) 0 a 0];
    else
        DH_params(2*i-1:2*i,:)=[(theta(2*i-1)*180/pi) 90 0 0; (theta(2*i)*180/pi) 0 a 0];
    end
end

% Calculate transformation matrix n_A_n+1 (A_wrt_prev) and store in cell
% array
A = cell(2*N,1);
for n=1:2*N
    theta_i=DH_params(n,1);
    alpha_i=DH_params(n,2);
    r_i=DH_params(n,3);
    d_i=DH_params(n,4);
    A{n}=[cosd(theta_i) -sind(theta_i)*cosd(alpha_i) sind(theta_i)*sind(alpha_i) r_i*cosd(theta_i);...
       sind(theta_i)  cosd(theta_i)*cosd(alpha_i) -cosd(theta_i)*sind(alpha_i) r_i*sind(theta_i);...
                  0              sind(alpha_i)   cosd(alpha_i)              d_i;...
                  0              0              0                         1];
end

% Create a list of transformation matrices wrt base for all joints
A_wrt_base=cell(2*N,1);
A_wrt_base{1}=A{1};
for n=2:2*N
    A_wrt_base{n}=A_wrt_base{n-1}*A{n};
end

for i=1:N
    for j=1:3*N
        M=floor((j-1)/3)+1;
        if j==1
           Td_prev=Td_0(j);
        end
        % Calculate delta and r
        if rem(i,2)==0
            delta_p=((120/(N+1))*(M)+120*(j-1)+87);
            delta_d=((120/(N+1))*(M)+120*(j-1)-3);
            r_p_j=[d-l_link; r*cosd(delta_p);r*sind(delta_p); 1];
            r_d_j=[-d;r*cosd(delta_d);r*sind(delta_d); 1];
        else
            delta_p=((120/(N+1))*(M)+120*(j-1)-3);
            delta_d=((120/(N+1))*(M)+120*(j-1)+87);
            if i==1
                L_d_prev=[-d;r*cosd(delta_d);r*sind(delta_d); 1];
                e_d_prev=L_d_prev(1:3)/norm(L_d_prev(1:3));
                e_d_0=e_d_prev;
                r_d_prev=[-d;r*cosd(delta_d);r*sind(delta_d); 1];
            end
            r_p_j=[d-l_link; r*sind(delta_p);-r*cosd(delta_p); 1];
            r_d_j=[-d;r*sind(delta_d);-r*cosd(delta_d); 1];
        end
        r_p{i,j}=r_p_j(1:3);
        r_d{i,j}=r_d_j(1:3);
        % Calculate L
        if i==1
            L_p=(A{2*i}*r_p_j)-(r_d_prev);
        else
            L_p=(A{2*i}*r_p_j)-(A{2*i-2}*r_d_prev);
        end
        L_d=A{2*i}*(r_d_j-r_p_j);
        % Calculate e
        e_p=L_p(1:3)/norm(L_p(1:3));
        e_d=L_d(1:3)/norm(L_d(1:3));
        % Calculate phi
        phi_p=acos(dot(e_p,e_d));
        phi_d=acos(dot(e_d_prev,e_p));
        % Get Tp
        T_p_j=Td_prev/(exp(mu*phi_d));
        T_p{i,j}=T_p_j*e_p;
        % Get Td
        T_d_j=T_p_j/(exp(mu*phi_p));
        T_d{i,j}=T_d_j*e_d;
        % Update prev values
        e_d_prev=e_d;
        r_d_prev=r_d_j;
        Td_prev=T_d_j;
    end
end

% Calculate F_cp and F_cd
for n=1:N
    for k=1:3*N
        M=floor((k-1)/3)+1;
        if (3*n+1 <= k) && (k<=3*N) && n<=M
            F_cp{n,k}=T_d{n,k}-T_p{n,k};
            if n==1
                F_cd{n,k}=T_p{n,k}-((tau_m(k)*r_drum/eta)*e_d_0);
            else
                F_cd{n,k}=T_p{n,k}-T_d{n-1,k};
            end
        end
        if (3*n-2 <= k) && (k <=3*n) && n==M
            F_cp{n,k}=-T_p{n,k};
        end
    end
end

% Calculate F_ec
for n=1:N
    F_ec_n=[0;0;0];
    A_2n=inv(A{2*n});
    R_2n=A_2n(1:3,1:3);
    for k=3*n+1:3*N
        F_ec_n=F_ec_n+((R_2n)*F_cd{n,k});
    end
    for k=3*n-2:3*N
        F_ec_n=F_ec_n+((R_2n)*F_cp{n,k});
    end
    F_ec(:,n)=F_ec_n;
end

% Calculate T_ec
for n=1:N
    T_ec_n=[0;0;0];
    A_2n=inv(A{2*n});
    R_2n=A_2n(1:3,1:3);
    for k=3*n+1:3*N
        T_ec_n=T_ec_n+cross((r_d{n,k}-P_link_cm),((R_2n)*F_cd{n,k}));
    end
    for k=3*n-2:3*N
        T_ec_n=T_ec_n+cross((r_p{n,k}-P_link_cm),((R_2n)*F_cp{n,k}));
    end
    T_ec(:,n)=T_ec_n;
end

== matlab function CDHRM_model_v1/Dynamic Model of the arm/M_inv(theta)/Newton-Euler Inverse Dynamics Block 17/Newton-Euler Recursive Inverse Dynamics Block ==
  data: theta input; u output; d_theta input; dd_theta input; m input; a input; d input; r input; g input; F_ec input; T_ec input
%% Neton-Euler Recursive Algorithm for Inverse Dynamics
function u  = fcn(theta, d_theta,dd_theta,m,a,d,r,g,F_ec,T_ec)
%% Parameters
N=9;
P_joint_to_joint=[a+2*d;0;0];
P_link_cm=[-(a/2+d);0;0];
z_0=[0;0;1];
x_0=[1;0;0];
% Create the D-H parameter table
DH_params=zeros(2*N,4);
for i=1:N
    if rem(i,2)==0
        DH_params(2*i-1:2*i,:)=[180+(theta(2*i-1)*180/pi) 90 0 0;...
                                180+(theta(2*i)*180/pi) 0 a 0];
    else
        DH_params(2*i-1:2*i,:)=[theta(2*i-1)*180/pi 90 0 0;...
                                theta(2*i)*180/pi 0 a 0];
    end
end
% Calculate transformation matrix n_A_n+1 (A_wrt_prev) and store in cell
% array
R = cell(2*N,1);
for n=1:2*N
    theta_i=DH_params(n,1);
    alpha_i=DH_params(n,2);
    R{n}=[cosd(theta_i) -sind(theta_i)*cosd(alpha_i) sind(theta_i)*sind(alpha_i);...
       sind(theta_i)  cosd(theta_i)*cosd(alpha_i) -cosd(theta_i)*sind(alpha_i);...
                  0              sind(alpha_i)   cosd(alpha_i) ];
end
% Calculate Inertia tensor
I = cell(N,1);
for i=1:N
    I{i}=[1/12*(m*(a)^2)+1/4*(m*r^2) 0 0;
                      0 1/12*(m*(a)^2)+1/4*(m*r^2) 0;
                      0 0 1/4*(m*r^2)];
end
%% Forward recursion
% Initialising the matrices
omega=zeros(3,N);
d_omega=zeros(3,N);
a_joint=zeros(3,N);
a_c=zeros(3,N);
% Initialising prev values
omega_prev=zeros(3,1);
d_omega_prev=zeros(3,1);
a_joint_prev=zeros(3,1);
for n=1:N
    omega(:,n)=(R{2*n-1}*R{2*n})'*(omega_prev + z_0*d_theta(2*n-1)) + ...
               (R{2*n})'*z_0*d_theta(2*n);
    d_omega(:,n)=(R{2*n-1}*R{2*n})'*(d_omega_prev + z_0*dd_theta(2*n-1)+...
                                     cross(omega(:,n),z_0*d_theta(2*n-1))) + ...
                 (R{2*n-1}*R{2*n})'*(cross((z_0*d_theta(2*n-1) + omega_prev),R{2*n-1}*z_0*d_theta(2*n))) + ...
                 (R{2*n})'*(z_0*dd_theta(2*n));
    if n==1
        a_joint(:,n)=[0;0;g];
    else
        a_joint(:,n)=(R{2*n-3}*R{2*n-2})'*a_joint_prev+ ...
                     cross(d_omega_prev,P_joint_to_joint)+...
                     cross(omega_prev,cross(omega_prev,P_joint_to_joint));
    end
    a_c(:,n)=(R{2*n-1}*R{2*n})'*a_joint(:,n)+...
             cross(d_omega(:,n),(P_joint_to_joint+P_link_cm))+...
             cross(omega(:,n),cross(omega(:,n),(P_joint_to_joint+P_link_cm)));
    % Update prev values for next iteration
    omega_prev=omega(:,n);
    d_omega_prev=d_omega(:,n);
    a_joint_prev=a_joint(:,n);
end

%% Backward recursion
% Initialising the matrices
F=zeros(3,N);
tau=zeros(3,N);
% Initialise next values
F_next=zeros(3,1);
tau_next=zeros(3,1);
for n=N:-1:1
   F(:,n) = F_next + m*a_c(:,n)-F_ec(:,n);
   tau(:,n) = tau_next - cross(F(:,n),(P_joint_to_joint+P_link_cm)) + ...
              cross(F_next,P_link_cm) + ...
              I{n}*d_omega(:,n)+ cross(omega(:,n),I{n}*omega(:,n))-T_ec(:,n);
   % Update next values for next iteration
   F_next=F(:,n);
   tau_next=tau(:,n);
end
%% Computing the output
u=vecnorm(tau)';
